simulink model "partitionedLifitngBdyForces_th"  (R2018b)
settings: Solver=VariableStepAuto  StartTime=0.0  StopTime=0  RelTol=1e-3
values from neighbouring files (symbols this model uses):
  angVelBdy = [0;0;0]    [partitionedLifitngBdy_ts.m]
  eulerAng = [0;0;0]    [partitionedLifitngBdy_ts.m]
  vCM = [0;0;0]    [partitionedLifitngBdy_ts.m]
  vFlow = [1;0;0.01]    [partitionedLifitngBdy_ts.m]
libraries: partitionedLifitngBdyForces_ul x1
settings Model: Creator=mcobb  LastModifiedBy=asiddiq2

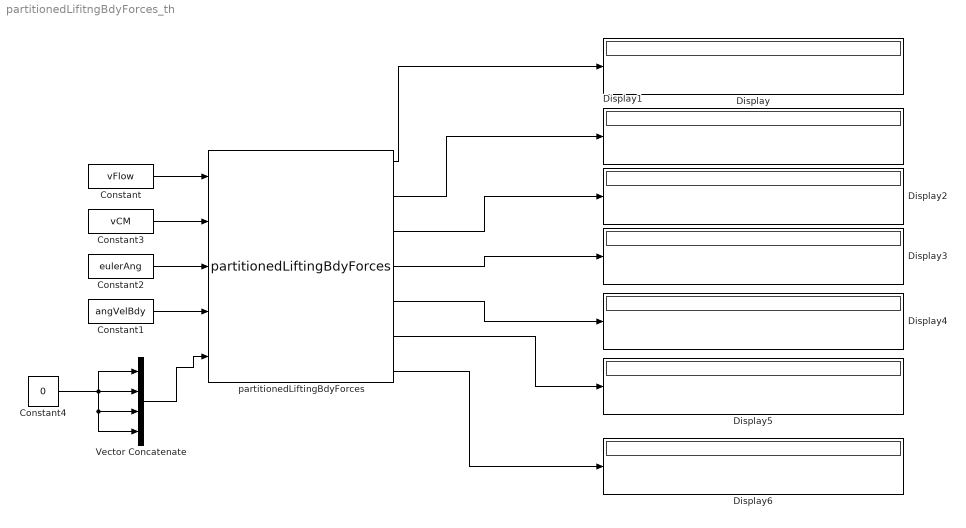
== system partitionedLifitngBdyForces_th ==
  Constant : Constant  Value=vFlow  VectorParams1D=off
  Constant1 : Constant  Value=angVelBdy  VectorParams1D=off
  Constant2 : Constant  Value=eulerAng  VectorParams1D=off
  Constant3 : Constant  Value=vCM  VectorParams1D=off
  Constant4 : Constant  Value=0
  Display{,1..6} (7 alike) : Display
  Vector Concatenate : Concatenate  NumInputs=4
  partitionedLiftingBdyForces : partitionedLifitngBdyForces_ul/partitionedLiftingBdyForces  rhoFluid=env.fluidDensity.Value  aeroCenterPos=vhcl.fluidMomentArms.Value  fluidRefArea=vhcl.fluidRefArea.Value  FluidStruct=vhcl.fluidCoeffData
  wires:
  Constant/1 -> partitionedLiftingBdyForces/1
  Constant1/1 -> partitionedLiftingBdyForces/4
  Constant2/1 -> partitionedLiftingBdyForces/3
  Vector Concatenate/1 -> partitionedLiftingBdyForces/5
  Constant4/1 -> Vector Concatenate/3, Vector Concatenate/4, Vector Concatenate/1, Vector Concatenate/2
  Constant3/1 -> partitionedLiftingBdyForces/2
  partitionedLiftingBdyForces/1 -> Display/1
  partitionedLiftingBdyForces/2 -> Display1/1
  partitionedLiftingBdyForces/3 -> Display2/1
  partitionedLiftingBdyForces/4 -> Display3/1
  partitionedLiftingBdyForces/7 -> Display6/1
  partitionedLiftingBdyForces/6 -> Display5/1
  partitionedLiftingBdyForces/5 -> Display4/1
